simulink model "Test_Stateflow"  (R2014a)
settings: Solver=FixedStepDiscrete  StartTime=0.0  StopTime=10.0  FixedStep=0.5  RelTol=1e-3
libraries: GPIO_Lib x4, STM32_Config_Lib x1
settings Model: Creator=jan  LastModifiedBy=jan
settings DataIOCC: LimitDataPoints=off
settings OptimizationCC: OptimizeModelRefInitCode=on  LifeSpan=1
settings HardwareCC: ProdLargestAtomicInteger=Integer  ProdLargestAtomicFloat=Float  ProdIntDivRoundTo=Zero  ProdEndianess=LittleEndian  ProdHWDeviceType=STMicroelectronics->STM32 32-bit Cortex-M
settings RTWCC: SystemTargetFile=stm32.tlc  TemplateMakefile=stm32.tmf  Description=stm32 (Embedded Target)  GenerateReport=on  ProcessScript=stm32_make_rtw_hook  Toolchain=Microsoft Visual C++ 2012 v11.0 | nmake (64-bit Windows)
settings CodeAppCC: IgnoreCustomStorageClasses=off  MaxIdLength=64  CustomSymbolStrType=$N$R$M  SimulinkBlockComments=off
settings STFCustomTargetCC: CodeReplacementLibrary=ARM CMSIS SIN COS  ParMdlRefBuildCompliant=on  ConcurrentExecutionCompliant=off  IncludeMdlTerminateFcn=off  GeneratePreprocessorConditionals=Use local settings  CombineOutputUpdateFcns=on  ERTCustomFileBanners=on  SupportContinuousTime=off  SupportNonInlinedSFcns=off  MATLABClassNameForMDSCustomization=Simulink.SoftwareTarget.ERTCustomization  GRTInterface=off  SystemTargetFile=stm32.tlc
settings ERTTargetCC: CodeReplacementLibrary=ARM CMSIS SIN COS  GenerateSampleERTMain=off  ParMdlRefBuildCompliant=on  IncludeMdlTerminateFcn=off  ERTSrcFileBannerTemplate=sourceFileTemplate.cgt  ERTHdrFileBannerTemplate=sourceFileTemplate.cgt  ERTDataSrcFileTemplate=sourceFileTemplate.cgt  ERTDataHdrFileTemplate=sourceFileTemplate.cgt  ERTCustomFileTemplate=customRoutineProcess.tlc

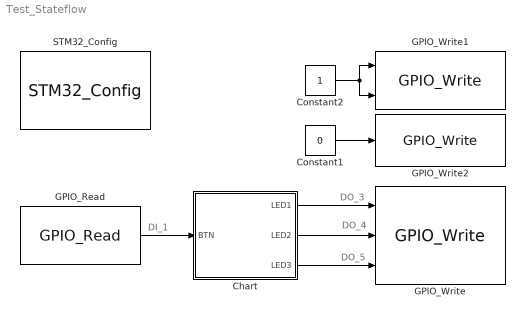
== system Test_Stateflow ==
  note: DI_1
  note: DO_5
  note: DO_4
  note: DO_3
  Chart : Stateflow chart  TreatAsAtomicUnit=on
  Constant1 : Constant  Value=0  OutDataTypeStr=uint8
  Constant2 : Constant  OutDataTypeStr=uint8
  GPIO_Read : GPIO_Lib/GPIO_Read  Port_name=GPIOE  Pin_0=off  Pin_1=off  Pin_2=off  Pin_3=off  Pin_4=off  Pin_5=off  Pin_6=off  Pin_7=off  Pin_8=on  Pin_9=off  Pin_10=off  Pin_11=off  Pin_12=off  Pin_13=off  Pin_14=off  Pin_15=off  PinList="GPIOA0  1GPIOE8   9  10  11  12  13  14  15"
  GPIO_Write : GPIO_Lib/GPIO_Write  Port_name=GPIOD  Pin0=off  Toggle_Pin0=off  Pin1=off  Toggle_Pin1=off  Pin2=off  Toggle_Pin2=off  Pin3=off  Toggle_Pin3=off  Pin4=off  Toggle_Pin4=off  Pin5=off  Toggle_Pin5=off  Pin6=off  Toggle_Pin6=off  Pin7=off  Toggle_Pin7=off  Pin8=off  Toggle_Pin8=off  Pin9=off  Toggle_Pin9=off  Pin10=off  Toggle_Pin10=off  Pin11=on  Toggle_Pin11=off  Pin12=on  Toggle_Pin12=off  Pin13=on  Toggle_Pin13=off  Pin14=off  Toggle_Pin14=off  Pin15=off  Toggle_Pin15=off  PinList="GPIOA7GPIOC4   5  11  13  14GPIOD0   1   7  11  12  13  14  15GPIOE1  3  4"
  GPIO_Write1 : GPIO_Lib/GPIO_Write  Port_name=GPIOC  Pin0=off  Toggle_Pin0=off  Pin1=off  Toggle_Pin1=off  Pin2=off  Toggle_Pin2=off  Pin3=off  Toggle_Pin3=off  Pin4=off  Toggle_Pin4=off  Pin5=off  Toggle_Pin5=off  Pin6=off  Toggle_Pin6=off  Pin7=off  Toggle_Pin7=off  Pin8=off  Toggle_Pin8=off  Pin9=off  Toggle_Pin9=off  Pin10=off  Toggle_Pin10=off  Pin11=off  Toggle_Pin11=off  Pin12=off  Toggle_Pin12=off  Pin13=on  Toggle_Pin13=off  Pin14=on  Toggle_Pin14=off  Pin15=off  Toggle_Pin15=off  PinList="GPIOA7GPIOC4   5  11  13  14GPIOD0   1   7  11  12  13  14  15GPIOE1  3  4"
  GPIO_Write2 : GPIO_Lib/GPIO_Write  Port_name=GPIOD  Pin0=off  Toggle_Pin0=off  Pin1=off  Toggle_Pin1=off  Pin2=off  Toggle_Pin2=off  Pin3=off  Toggle_Pin3=off  Pin4=off  Toggle_Pin4=off  Pin5=off  Toggle_Pin5=off  Pin6=off  Toggle_Pin6=off  Pin7=on  Toggle_Pin7=off  Pin8=off  Toggle_Pin8=off  Pin9=off  Toggle_Pin9=off  Pin10=off  Toggle_Pin10=off  Pin11=off  Toggle_Pin11=off  Pin12=off  Toggle_Pin12=off  Pin13=off  Toggle_Pin13=off  Pin14=off  Toggle_Pin14=off  Pin15=off  Toggle_Pin15=off  PinList="GPIOA7GPIOC4   5  11  13  14GPIOD0   1   7  11  12  13  14  15GPIOE1  3  4"
  STM32_Config : STM32_Config_Lib/STM32_Config  Priority=0  Project_Path=E:\HTWAA_car_32b\projects\Test_Stateflow\  Config_File=HTWAA_32b.ioc  MCU_Name=STM32F429VITx
  wires:
  Constant2/1 -> GPIO_Write1/2, GPIO_Write1/1
  Constant1/1 -> GPIO_Write2/1
  Chart/1(LED1) -> GPIO_Write/1
  Chart/2(LED2) -> GPIO_Write/2
  Chart/3(LED3) -> GPIO_Write/3
  GPIO_Read/1 -> Chart/1(BTN)

== stateflow chart Test_Stateflow/Chart ==
  state S1
    en: LED1 = 1;
    en: LED2 = 0;
    en: LED3 = 0;
  state S2
    en: LED1 = 0;
    en: LED2 = 1;
    en: LED3 = 0;
  state S3
    en: LED1 = 0;
    en: LED2 = 0;
    en: LED3 = 1;
  (default) -> S1
  S1 -> S2 : [BTN == 1]
  S3 -> S1 : after(2, sec)
  S2 -> S3 : [BTN == 0]
  data: BTN input; LED1 output; LED2 output; LED3 output
